simulink model "Chua_TxRx_final_post"  (R2020a)
settings: Solver=VariableStepAuto  StartTime=0.0  StopTime=300  RelTol=1e-3
libraries: simulink x1
settings Model: Creator=RaviM  LastModifiedBy=RaviM

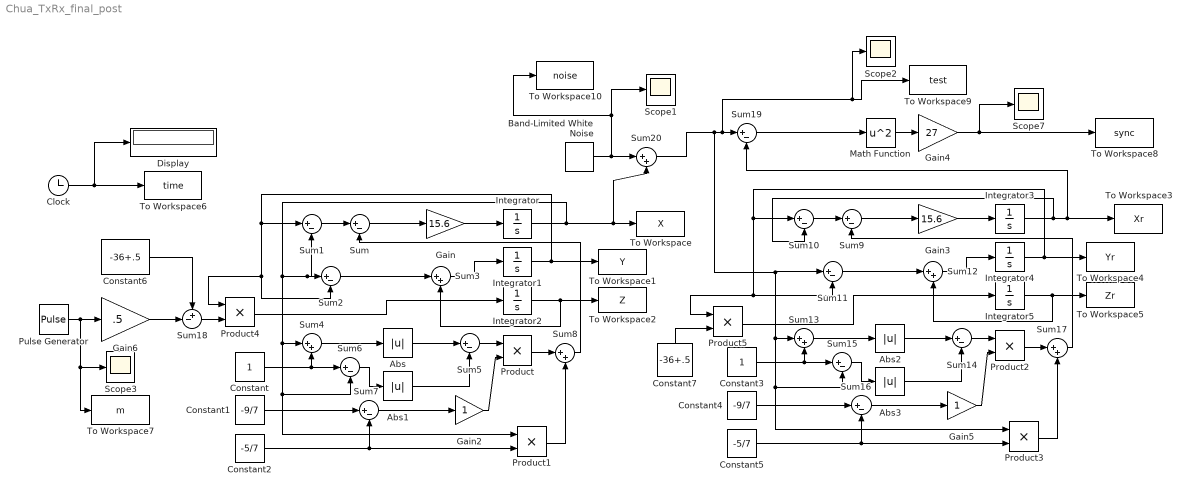
== system Chua_TxRx_final_post ==
  Abs{,1..3} (4 alike) : Abs
  Band-Limited White Noise : simulink/Sources/Band-Limited White Noise  Cov=[0.03]  Ts=1  seed=[233]
  Clock : Clock
  Constant : Constant
  Constant1 : Constant  Value=-9/7
  Constant2 : Constant  Value=-5/7
  Constant3 : Constant
  Constant4 : Constant  Value=-9/7
  Constant5 : Constant  Value=-5/7
  Constant6 : Constant  Value=-36+.5
  Constant7 : Constant  Value=-36+.5
  Display : Display
      settings: Decimation=5
  Gain : Gain  Gain=15.6
  Gain2 : Gain
  Gain3 : Gain  Gain=15.6
  Gain4 : Gain  Gain=27
  Gain5 : Gain
  Gain6 : Gain  Gain=.5
  Integrator{,1..5} (6 alike) : Integrator  InitialCondition=0.1
  Math Function : Math  Operator=square  SignedPower=on  SaturateOnIntegerOverflow=on
  Product{,1..5} (6 alike) : Product
  Pulse Generator : DiscretePulseGenerator  PulseType=Time based  Amplitude=5  Period=100  PulseWidth=50  PhaseDelay=50
  Scope{1..3,7} (4 alike) : Scope
  Sum{,1..2,5..7,9..11,14..16,19} (13 alike) : Sum  Inputs=|+-
  Sum{3..4,8,12..13,17,20} (7 alike) : Sum  Inputs=|++
  Sum18 : Sum  Inputs=+-|
  To Workspace : ToWorkspace  VariableName=X  SaveFormat=Timeseries  SampleTime=-1
  To Workspace1 : ToWorkspace  VariableName=Y  SaveFormat=Timeseries  SampleTime=-1
  To Workspace10 : ToWorkspace  VariableName=noise  SampleTime=-1
  To Workspace2 : ToWorkspace  VariableName=Z  SaveFormat=Timeseries  SampleTime=-1
  To Workspace3 : ToWorkspace  VariableName=Xr  SaveFormat=Timeseries  SampleTime=-1
  To Workspace4 : ToWorkspace  VariableName=Yr  SaveFormat=Timeseries  SampleTime=-1
  To Workspace5 : ToWorkspace  VariableName=Zr  SaveFormat=Timeseries  SampleTime=-1
  To Workspace6 : ToWorkspace  VariableName=time  SampleTime=-1
  To Workspace7 : ToWorkspace  VariableName=m  SampleTime=-1
  To Workspace8 : ToWorkspace  VariableName=sync  SampleTime=-1
  To Workspace9 : ToWorkspace  VariableName=test  SampleTime=-1
  wires:
  Sum5/1 -> Product/1
  Product4/1 -> Integrator2/1
  Sum3/1 -> Integrator1/1
  Gain2/1 -> Product/2
  Abs1/1 -> Sum5/2
  Sum2/1 -> Sum3/1
  Constant1/1 -> Sum7/1
  Gain/1 -> Integrator/1
  Constant/1 -> Sum6/1, Sum4/2
  Abs/1 -> Sum5/1
  Sum1/1 -> Sum/1
  Product/1 -> Sum8/1
  Product1/1 -> Sum8/2
  Sum6/1 -> Abs1/1
  Sum4/1 -> Abs/1
  Constant2/1 -> Product1/2, Sum7/2
  Sum8/1 -> Sum/2
  Sum7/1 -> Gain2/1
  Integrator2/1 -> Sum3/2, To Workspace2/1
  Sum/1 -> Gain/1
  Sum14/1 -> Product2/1
  Product5/1 -> Integrator5/1
  Sum12/1 -> Integrator4/1
  Gain5/1 -> Product2/2
  Abs3/1 -> Sum14/2
  Sum11/1 -> Sum12/1
  Constant4/1 -> Sum16/1
  Gain3/1 -> Integrator3/1
  Constant3/1 -> Sum15/1, Sum13/2
  Abs2/1 -> Sum14/1
  Sum10/1 -> Sum9/1
  Product2/1 -> Sum17/1
  Product3/1 -> Sum17/2
  Sum15/1 -> Abs3/1
  Sum13/1 -> Abs2/1
  Constant5/1 -> Product3/2, Sum16/2
  Sum17/1 -> Sum9/2
  Sum16/1 -> Gain5/1
  Integrator5/1 -> Sum12/2, To Workspace5/1
  Sum9/1 -> Gain3/1
  Constant6/1 -> Sum18/1
  Sum18/1 -> Product4/2
  Pulse Generator/1 -> Gain6/1, Scope3/1, To Workspace7/1
  Gain6/1 -> Sum18/2
  Clock/1 -> Display/1, To Workspace6/1
  Integrator1/1 -> Sum2/2, Product4/1, Sum1/1, To Workspace1/1
  Integrator4/1 -> Sum11/2, Product5/1, Sum10/1, To Workspace4/1
  Constant7/1 -> Product5/2
  Gain4/1 -> Scope7/1, To Workspace8/1
  Integrator3/1 -> To Workspace3/1, Sum19/2, Sum10/2
  Math Function/1 -> Gain4/1
  Integrator/1 -> Product1/1, Sum6/2, Sum4/1, Sum1/2, Sum2/1, To Workspace/1, Sum20/2
  Band-Limited White Noise/1 -> To Workspace10/1, Scope1/1, Sum20/1
  Sum19/1 -> Math Function/1
  Sum20/1 -> Sum11/1, Sum13/1, Product3/1, Sum15/2, Scope2/1, To Workspace9/1, Sum19/1
